simulink model "modulation"  (R2022b)
settings: Solver=VariableStepAuto  StartTime=0.0  StopTime=1  RelTol=1e-3
libraries: dspsrcs4 x3, dsparch4 x2
settings Model: Creator=osama  LastModifiedBy=osama

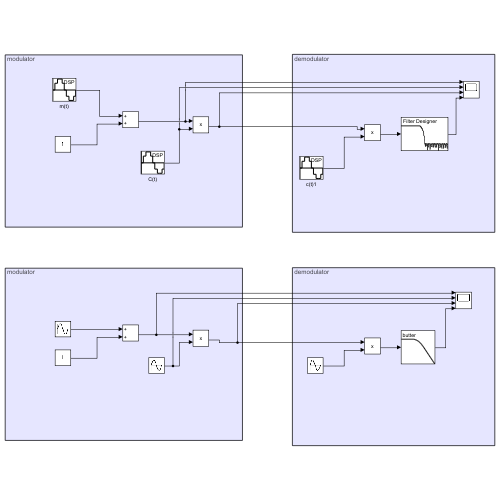
[thumbnail: Simulink's stored preview of the top-level diagram]
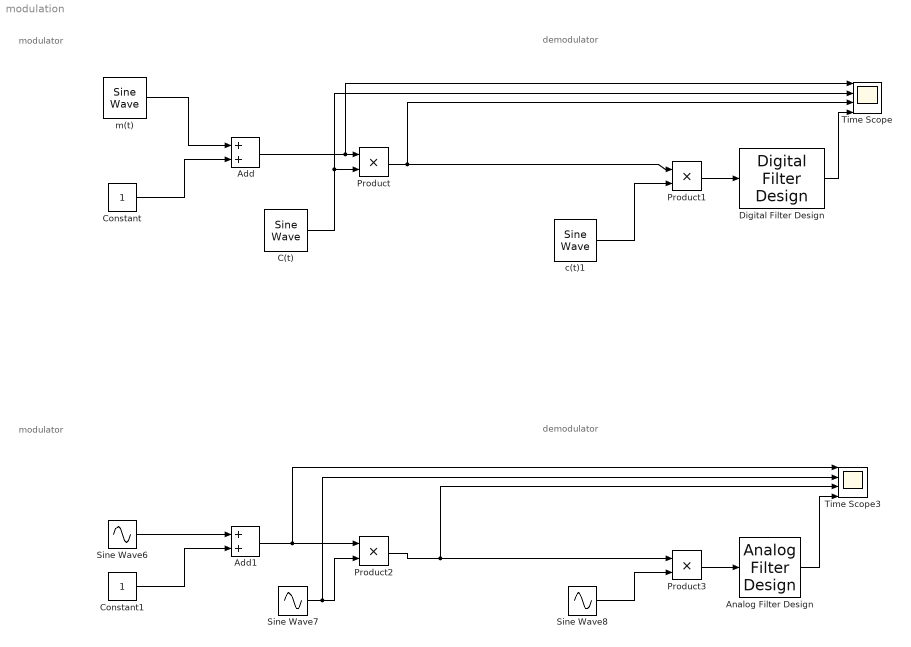
== system modulation ==
  note: demodulator
  note: modulator
  note: demodulator
  note: modulator
  Add : Sum
  Add1 : Sum
  Analog Filter Design : dsparch4/Analog Filter Design  method=Butterworth  filttype=Lowpass  N=2  Wlo=2*pi*8000  Whi=80  Rp=2  Rs=40
  C(t) : dspsrcs4/Sine Wave  Amplitude=1  Frequency=100000  Phase=0  SampleMode=Discrete  OutComplex=Real  CompMethod=Trigonometric fcn  TableSize=Speed  SampleTime=1/900000  SamplesPerFrame=1  ResetState=Restart at time zero  OutputFrames=off  dataType=double  wordLen=16  udDataType=sfix(16)  fracBitsMode=Best precision  numFracBits=15  OutDataTypeStr=double  LastOutDataTypeStr=double
  Constant : Constant
  Constant1 : Constant
  Digital Filter Design : dsparch4/Digital Filter Design  mwdsp_browser_bugfix_var=off
  Product{,1..3} (4 alike) : Product
  Sine Wave6 : Sin  Amplitude=0.9  Frequency=2*pi*8000  SampleTime=0
  Sine Wave7 : Sin  Frequency=2*pi*100000  SampleTime=0
  Sine Wave8 : Sin  Frequency=2*pi*100000  SampleTime=0
  Time Scope : Scope  NumInputPorts=4
  Time Scope3 : Scope  NumInputPorts=4
  c(t)1 : dspsrcs4/Sine Wave  Amplitude=1  Frequency=100000  Phase=0  SampleMode=Discrete  OutComplex=Real  CompMethod=Trigonometric fcn  TableSize=Speed  SampleTime=1/900000  SamplesPerFrame=1  ResetState=Restart at time zero  OutputFrames=off  dataType=double  wordLen=16  udDataType=sfix(16)  fracBitsMode=Best precision  numFracBits=15  OutDataTypeStr=double  LastOutDataTypeStr=double
  m(t) : dspsrcs4/Sine Wave  Amplitude=0.9  Frequency=8000  Phase=0  SampleMode=Discrete  OutComplex=Real  CompMethod=Trigonometric fcn  TableSize=Speed  SampleTime=1/300000  SamplesPerFrame=1  ResetState=Restart at time zero  OutputFrames=off  dataType=double  wordLen=16  udDataType=sfix(16)  fracBitsMode=Best precision  numFracBits=15  OutDataTypeStr=double  LastOutDataTypeStr=double
  wires:
  m(t)/1 -> Add/1
  Constant/1 -> Add/2
  Add/1 -> Time Scope/1, Product/1
  C(t)/1 -> Time Scope/2, Product/2
  Product/1 -> Time Scope/3, Product1/1
  c(t)1/1 -> Product1/2
  Product1/1 -> Digital Filter Design/1
  Sine Wave8/1 -> Product3/2
  Product2/1 -> Time Scope3/3, Product3/1
  Constant1/1 -> Add1/2
  Product3/1 -> Analog Filter Design/1
  Analog Filter Design/1 -> Time Scope3/4
  Sine Wave7/1 -> Time Scope3/2, Product2/2
  Add1/1 -> Time Scope3/1, Product2/1
  Sine Wave6/1 -> Add1/1
  Digital Filter Design/1 -> Time Scope/4
